simulink subsystem "startQuat2MRP"  (R2021a)
settings: Solver=VariableStepAuto  StartTime=0.0  StopTime=10.0  RelTol=1e-3
settings Model: Creator=noraw  LastModifiedBy=noraw

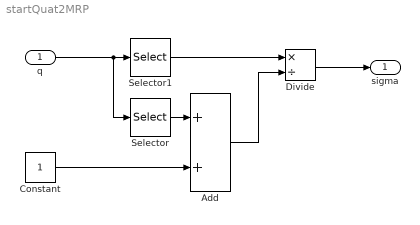
== system startQuat2MRP ==
  q : Inport
  Add : Sum
  Constant : Constant
  Divide : Product  Inputs=*/
  Selector : Selector  InputPortWidth=4  IndexOptions=Index vector (dialog)  Indices=[1]  OutputSizes=1
  Selector1 : Selector  InputPortWidth=4  IndexOptions=Index vector (dialog)  Indices=[2 3 4]  OutputSizes=1
  sigma : Outport
  wires:
  Selector1/1 -> Divide/1
  Add/1 -> Divide/2
  Divide/1 -> sigma/1
  Selector/1 -> Add/1
  q/1 -> Selector1/1, Selector/1
  Constant/1 -> Add/2
